simulink model "RLC_embedded_coder"  (R2022b)
settings: Solver=FixedStepDiscrete  StartTime=0.0  StopTime=Inf  RelTol=1e-3
InitFcn:
  | parametri_embedded
undefined symbols (not defined in the file): ADC_gain, current_gain, current_offset, data_size, DiscIntNeverNeededParam, Down, GPTRIP1SEL, GPTRIP2SEL, i_max, Kd_u, Ki_i, Ki_u, Kp_i, Kp_u, offset_filter, PWM_PERIOD, ref_counter_cmpr, ref_counter_prd, ref_value_high, ref_value_low, SAMPLE_FREQ, SAMPLE_TIME, tau, TZ1, TZ2, u_max, Up, voltage_gain, voltage_offset
libraries: simulink x9, c2802xlib x3, c280xlib x2, c2000lib x1, c2806xlib x1
settings Model: SimulationMode=external  ExtModeTrigDuration=8  Creator=Jan  LastModifiedBy=Jan
settings SolverCC: ZeroCrossAlgorithm=Adaptive  AutoInsertRateTranBlk=on
settings DataIOCC: ReturnWorkspaceOutputs=off
settings OptimizationCC: UseDivisionForNetSlopeComputation=on  GainParamInheritBuiltInType=on  UseFloatMulNetSlope=on  DefaultUnderspecifiedDataType=single  PassReuseOutputArgsAs=Individual arguments  NoFixptDivByZeroProtection=on  EfficientFloat2IntCast=on  LifeSpan=1  MaxStackSize=1024  OptimizeBlockOrder=speed  DifferentSizesBufferReuse=on  DenormalBehavior=FlushToZero  EfficientTunableParamExpr=on
settings DebuggingCC: IgnoredZcDiagnostic=none  ParameterTunabilityLossMsg=error
settings HardwareCC: ProdBitPerChar=16  ProdBitPerInt=16  ProdBitPerPointer=32  ProdBitPerSizeT=32  ProdBitPerPtrDiffT=32  ProdLargestAtomicInteger=Integer  ProdLargestAtomicFloat=None  ProdWordSize=16  ProdLongLongMode=on  ProdHWDeviceType=Texas Instruments->C2000
settings SFSimCC: MATLABDynamicMemAlloc=off
settings RTWCC: Description=Embedded Coder  SystemTargetFile=ert.tlc  HardwareBoard=TI Piccolo F28069M LaunchPad  TLCOptions=-aInlineSetEventsForThisBaseRateFcn=TLC_FALSE -aSuppressMultiTaskScheduler=TLC_FALSE -aRateBasedStepFcn=1  TemplateMakefile=ert_default_tmf  Toolchain=Texas Instruments Code Composer Studio (C2000)
settings CodeAppCC: ForceParamTrailComments=on  IgnoreCustomStorageClasses=off  OperatorAnnotations=on  SimulinkDataObjDesc=on  SFDataObjDesc=on  CustomSymbolStrGlobalVar=rt$N$M  CustomSymbolStrType=$N$M  CustomSymbolStrFcn=$N$M$F  CustomSymbolStrMacro=$N$M  InsertBlockDesc=on
settings ERTTargetCC: CodeReplacementLibrary=TI C28x  IncludeMdlTerminateFcn=off  CombineSignalStateStructs=on  SupportComplex=off  SupportNonInlinedSFcns=on  ExtModeTransport=4  ExtModeStaticAlloc=on  ExtModeAutomaticAllocSize=off  ExtModeMexFile=ext_xcp  ExtModeIntrfLevel=Level2 - Open  ERTFilePackagingFormat=CompactWithDataFile

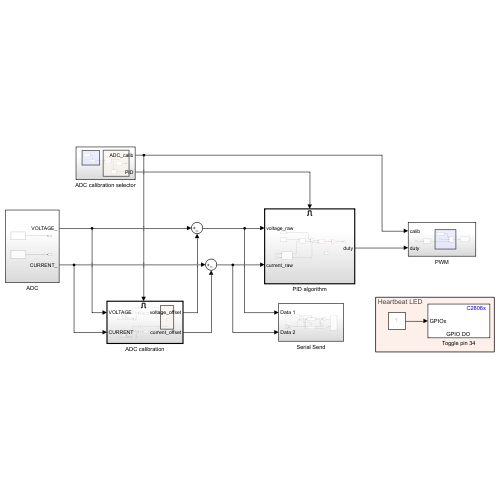
[thumbnail: Simulink's stored preview of the top-level diagram]
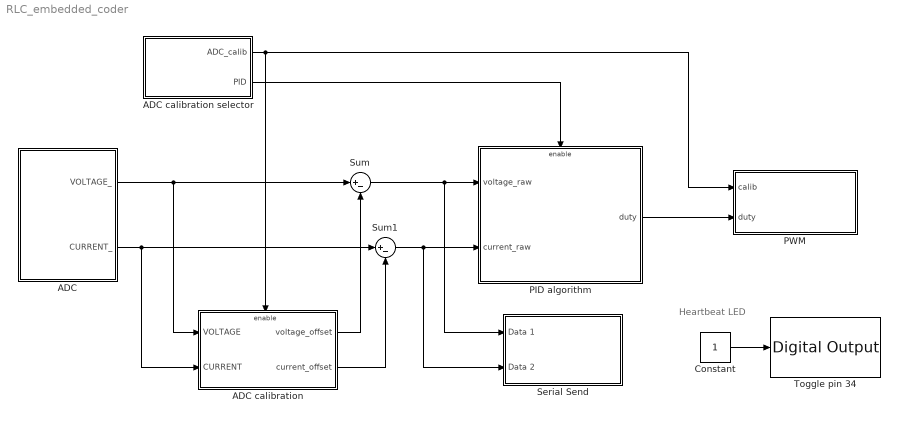
== system RLC_embedded_coder ==
  note: Heartbeat LED
  ADC : Subsystem
  ADC calibration : Subsystem
  ADC calibration selector : Subsystem
  Constant : Constant  SampleTime=0.7
  PID algorithm : Subsystem
  PWM : Subsystem
  Serial Send : Subsystem
  Sum : Sum  Inputs=|+-  OutDataTypeStr=Inherit: Same as first input
  Sum1 : Sum  Inputs=|+-  OutDataTypeStr=Inherit: Same as first input
  Toggle pin 34 : c2806xlib/Digital Output  GPIO_Number=GPIO32~GPIO39  GPIO_Bit0=off  GPIO_BIT0_Toggle=off  GPIO_Bit1=off  GPIO_BIT1_Toggle=off  GPIO_Bit2=on  GPIO_BIT2_Toggle=on  GPIO_Bit3=off  GPIO_BIT3_Toggle=off  GPIO_Bit4=off  GPIO_BIT4_Toggle=off  GPIO_Bit5=off  GPIO_BIT5_Toggle=off  GPIO_Bit6=off  GPIO_BIT6_Toggle=off  GPIO_Bit7=off  GPIO_BIT7_Toggle=off
  wires:
  Constant/1 -> Toggle pin 34/1
  ADC/2(CURRENT_) -> ADC calibration/2(CURRENT), Sum1/1
  ADC calibration selector/2(PID) -> PID algorithm/Enable
  Sum/1 -> Serial Send/1(Data 1), PID algorithm/1(voltage_raw)
  Sum1/1 -> PID algorithm/2(current_raw), Serial Send/2(Data 2)
  ADC/1(VOLTAGE_) -> ADC calibration/1(VOLTAGE), Sum/1
  PID algorithm/1(duty) -> PWM/2(duty)
  ADC calibration/1(voltage_offset) -> Sum/2
  ADC calibration/2(current_offset) -> Sum1/2
  ADC calibration selector/1(ADC_calib) -> PWM/1(calib), ADC calibration/Enable

== system RLC_embedded_coder/ADC ==
  note: ADC
  CURRENT : c2802xlib/ADC  blkParamProc=C2000  ADCModule=1  samplingMode=Single sample mode  ADCResolution=12-bit (Single-ended input)  useSOC1=SOC2  useSOC2=SOC0_SOC1  SOCAcquisitionWindow=7  SOCTriggerSource=ePWM1_ADCSOCA  SOCInterruptTrigger=No ADCINT  Ts=SAMPLE_TIME  dType=int16  postInterrupt=on  interruptSel=ADCINT1  ADCINTContinuous=off  endma=off  chdma=1  conv1=ADCINA0  conv2=ADCINA0 and ADCINB0  conv1_Type4=ADCIN0  conv2_Type4=ADCIN0 and ADCIN1
      settings: LibrarySourceBlock=c2806xlib/ADC
  VOLTAGE : c2802xlib/ADC  blkParamProc=C2000  ADCModule=1  samplingMode=Single sample mode  ADCResolution=12-bit (Single-ended input)  useSOC1=SOC1  useSOC2=SOC0_SOC1  SOCAcquisitionWindow=7  SOCTriggerSource=ePWM1_ADCSOCA  SOCInterruptTrigger=No ADCINT  Ts=SAMPLE_TIME  dType=int16  postInterrupt=off  interruptSel=ADCINT1  ADCINTContinuous=off  endma=off  chdma=1  conv1=ADCINA1  conv2=ADCINA0 and ADCINB0  conv1_Type4=ADCIN0  conv2_Type4=ADCIN0 and ADCIN1
      settings: LibrarySourceBlock=c2806xlib/ADC
  VOLTAGE_ : Outport
  CURRENT_ : Outport  Port=2
  wires:
  VOLTAGE/1 -> VOLTAGE_/1
  CURRENT/1 -> CURRENT_/1

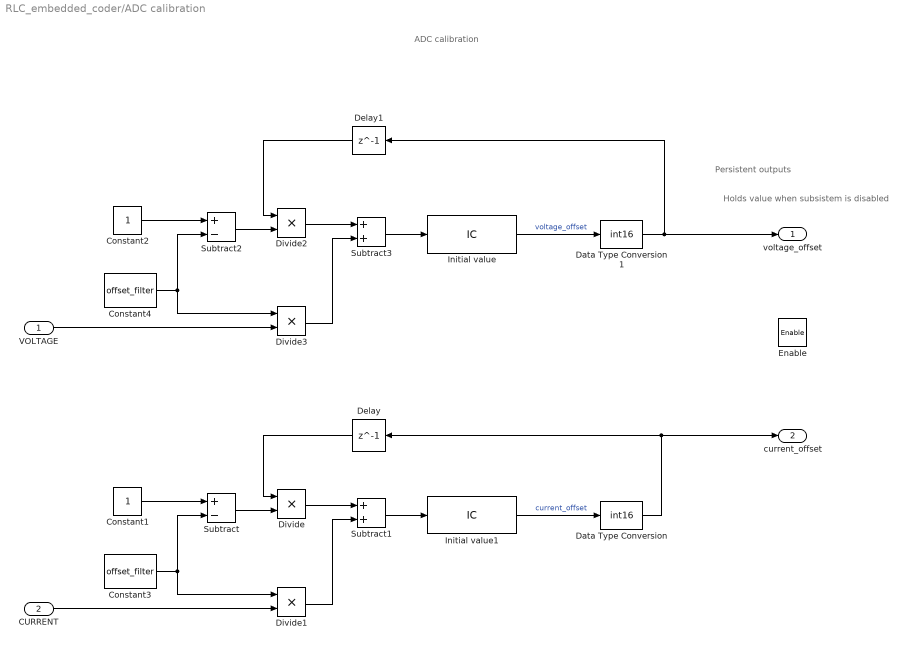
== system RLC_embedded_coder/ADC calibration ==
  note: Holds value when subsistem is disabled
  note: Persistent outputs
  note: ADC calibration
  VOLTAGE : Inport
  CURRENT : Inport  Port=2
  Enable : EnablePort
  Constant1 : Constant
  Constant2 : Constant
  Constant3 : Constant  Value=offset_filter
  Constant4 : Constant  Value=offset_filter
  Data Type Conversion : DataTypeConversion  OutDataTypeStr=int16  SaturateOnIntegerOverflow=off  RndMeth=Floor
  Data Type Conversion1 : DataTypeConversion  OutDataTypeStr=int16  SaturateOnIntegerOverflow=off  RndMeth=Floor
  Delay : Delay  DelayLength=1
  Delay1 : Delay  DelayLength=1
  Divide{,1..3} (4 alike) : Product  Inputs=**
  Initial value : InitialCondition  Value=voltage_offset
  Initial value1 : InitialCondition  Value=current_offset
  Subtract : Sum  Inputs=+-
  Subtract1 : Sum
  Subtract2 : Sum  Inputs=+-
  Subtract3 : Sum
  voltage_offset : Outport  OutDataTypeStr=int16
  current_offset : Outport  Port=2  OutDataTypeStr=int16
  wires:
  Subtract/1 -> Divide/2
  CURRENT/1 -> Divide1/2
  Constant3/1 -> Subtract/2, Divide1/1
  Constant1/1 -> Subtract/1
  Divide/1 -> Subtract1/1
  Divide1/1 -> Subtract1/2
  Delay/1 -> Divide/1
  Data Type Conversion/1 -> current_offset/1, Delay/1
  Delay1/1 -> Divide2/1
  Divide3/1 -> Subtract3/2
  Constant2/1 -> Subtract2/1
  VOLTAGE/1 -> Divide3/2
  Divide2/1 -> Subtract3/1
  Constant4/1 -> Subtract2/2, Divide3/1
  Subtract2/1 -> Divide2/2
  Initial value/1 -> Data Type Conversion1/1  "voltage_offset"
  Subtract3/1 -> Initial value/1
  Data Type Conversion1/1 -> voltage_offset/1, Delay1/1
  Subtract1/1 -> Initial value1/1
  Initial value1/1 -> Data Type Conversion/1  "current_offset"

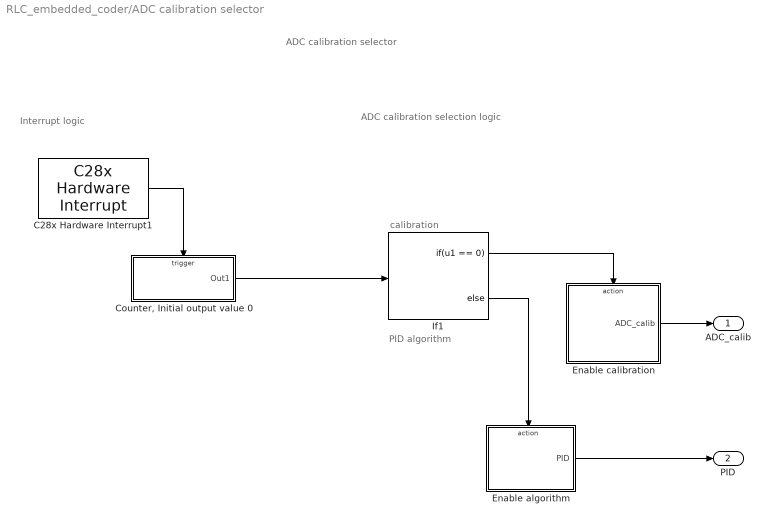
== system RLC_embedded_coder/ADC calibration selector ==
  note: calibration
  note: ADC calibration selection logic
  note: Interrupt logic
  note: PID algorithm
  note: ADC calibration selector
  C28x Hardware Interrupt1 : c2000lib/Scheduling/C28x Hardware Interrupt  irqnumbers=1  pienumbers=4  irqpriorities=30  irqpreempts=1  showinput=off  dspchiptype=C280X
  "Counter, Initial output value 0" : Subsystem  TreatAsAtomicUnit=on
  Enable algorithm : Subsystem  TreatAsAtomicUnit=on
  Enable calibration : Subsystem  TreatAsAtomicUnit=on
  If1 : If  IfExpression=u1 == 0
  ADC_calib : Outport
  PID : Outport  Port=2
  wires:
  If1/1 -> Enable calibration/Action
  If1/2 -> Enable algorithm/Action
  Enable algorithm/1(PID) -> PID/1
  Enable calibration/1(ADC_calib) -> ADC_calib/1
  C28x Hardware Interrupt1/1 -> "Counter, Initial output value 0"/Trigger
  "Counter, Initial output value 0"/1(Out1) -> If1/1

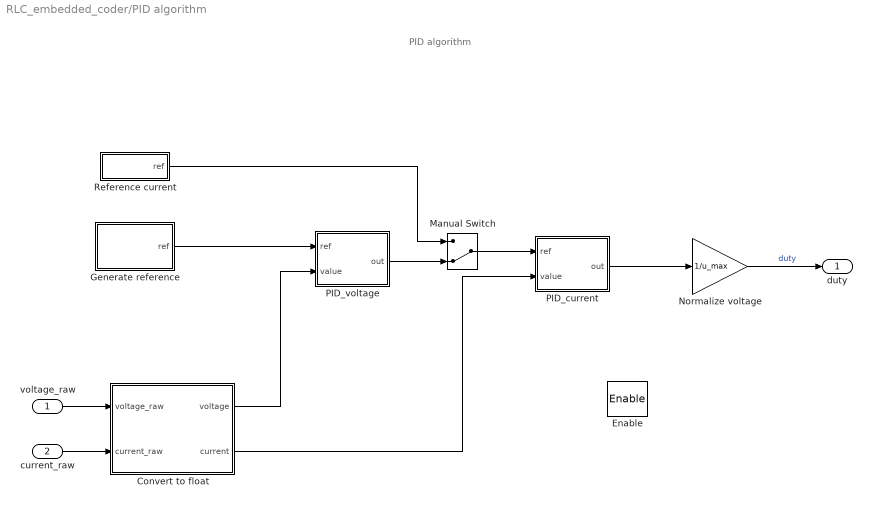
== system RLC_embedded_coder/PID algorithm ==
  note: PID algorithm
  voltage_raw : Inport
  current_raw : Inport  Port=2
  Enable : EnablePort
  Convert to float : Subsystem
  Generate reference : Subsystem
  Manual Switch : ManualSwitch  CurrentSetting=0
  Normalize voltage : Gain  Gain=1/u_max
  PID_current : Subsystem  mask{Kp=Kp_i, Ki=Ki_i, Kd=0, tau=0, lim=u_max, SAMPLE_TIME=SAMPLE_TIME}
      mask prompts: Kp "Proportional Gain"; Ki "Integral Gain"; Kd "Derivative Gain"; tau "Derivative filter"; lim "Output Limit"; SAMPLE_TIME "Sample Time"
      mask DialogControl DescTextVar Prompt: Discrete PID controller with D term filtering
  PID_voltage : Subsystem  mask{Kp=Kp_u, Ki=Ki_u, Kd=Kd_u, tau=tau, lim=i_max, SAMPLE_TIME=SAMPLE_TIME}
      mask prompts: Kp "Proportional Gain"; Ki "Integral Gain"; Kd "Derivative Gain"; tau "Derivative filter"; lim "Output Limit"; SAMPLE_TIME "Sample Time"
      mask DialogControl DescTextVar Prompt: Discrete PID controller with D term filtering
  Reference current : Subsystem
  duty : Outport
  wires:
  Generate reference/1(ref) -> PID_voltage/1(ref)
  Reference current/1(ref) -> Manual Switch/1
  Manual Switch/1 -> PID_current/1(ref)
  PID_voltage/1(out) -> Manual Switch/2
  PID_current/1(out) -> Normalize voltage/1
  Normalize voltage/1 -> duty/1  "duty"
  voltage_raw/1 -> Convert to float/1(voltage_raw)
  current_raw/1 -> Convert to float/2(current_raw)
  Convert to float/1(voltage) -> PID_voltage/2(value)
  Convert to float/2(current) -> PID_current/2(value)

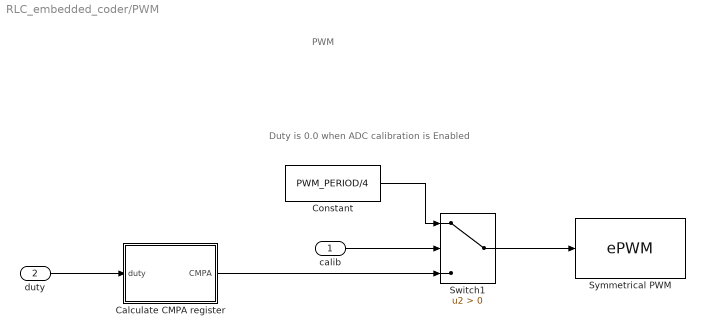
== system RLC_embedded_coder/PWM ==
  note: Duty is 0.0 when ADC calibration is Enabled
  note: PWM
  calib : Inport
  duty : Inport  Port=2
  Calculate CMPA register : Subsystem
  Constant : Constant  Value=PWM_PERIOD/4  SampleTime=-1
  Switch1 : Switch  Criteria=u2 > Threshold  SaturateOnIntegerOverflow=off  InputSameDT=off
  Symmetrical PWM : c2802xlib/ePWM  PwmType=C2000  useModule=ePWM1  ePWMxLINKTBPRD=Not Linked  periodUnits=Clock cycles  timerSource=Specify via dialog  timerPeriod_clk=int32(PWM_PERIOD/2)  timerPeriod_sec=0.0001  tbshadow=Counter equals to zero  countingMode=Up-Down  phaseActiveEnable=Disable  phaseDirection=Count down after sync  phaseActive=0  synchronizationEnable=off  dcaevt1Sync=off  dcbevt1Sync=off  synchronizationOption=Disable  dcbevt1SyncOut=off  dcaevt1SyncOut=off  cmpdSyncOut=off  cmpcSyncOut=off  cmpbSyncOut=off  zeroSyncOut=off  swfSyncOut=off  perSynchronizationOption=Counter equals to period (CTR=PRD)  clockPrescale=1  HSclockPrescale=1  enswap=off  ePWMxAStatus=on  ePWMxAactionLogic1=Do nothing  ePWMxAactionLogic2=Do nothing  ePWMxAactionLogic3=Set  ePWMxAactionLogic4=Clear  ePWMxAactionLogic5=Do nothing  ePWMxAactionLogic6=Do nothing  ePWMxACSFenable=off  ePWMxACSFvalue=Forcing disable  ePWMxASFreload=Zero  ePWMxBStatus=on  ePWMxBactionLogic1=Do nothing  ePWMxBactionLogic2=Do nothing  ePWMxBactionLogic3=Clear  ePWMxBactionLogic4=Set  ePWMxBactionLogic5=Do nothing  ePWMxBactionLogic6=Do nothing  ePWMxBCSFenable=off  ePWMxBCSFvalue=Forcing disable  ePWMxBSFreload=Zero  ePWNxBOutWay=on  ePWMxLINKCMPA=Not Linked  CMPAUnits=Clock cycles  CMPASource=Input port  CMPAValue_per=0  CMPAValue_clk=0  enCMPAshadow=Counter equals to zero (CTR=Zero)  ePWMxLINKCMPB=Not Linked  CMPBUnits=Clock cycles  CMPBSource=Specify via dialog  CMPBValue_per=0  CMPBValue_clk=0  enCMPBshadow=Counter equals to zero (CTR=Zero)  ePWMxLINKCMPC=Not Linked  CMPCUnits=Clock cycles  CMPCSource=Specify via dialog  CMPCValue_per=50  CMPCValue_clk=32000  enCMPCshadow=Counter equals to zero (CTR=Zero)  ePWMxLINKCMPD=Not Linked  CMPDUnits=Clock cycles  CMPDSource=Specify via dialog  CMPDValue_per=50  CMPDValue_clk=32000  enCMPDshadow=Counter equals to zero (CTR=Zero)  enableDBePWMxA=off  enableDBePWMxB=off  enhalfcycle=off  DBpolarity=Active high (AH)  DBedgeDelay=Positive  DBSource_ePWMxA=ePWMxA  DBSource_ePWMxB=ePWMxA  DBPeriodUnits=Clock cycles  DBperiodSource=Specify via dialog  REDperiod=0  FEDperiod=0  REDperiod_sec=0  FEDperiod_sec=0  LoadModeDBRED=Immediate without using shadow  LoadModeDBFED=Immediate without using shadow  adcstartModuleA=on  adcrequestEventA=First event  adcstartEventA=Counter equals to zero (CTR=Zero)  adcstartEventA_type2=Digital Compare Module A Event 1 start of conversion (DCAEVT1.soc)  adcstartModuleB=off  adcrequestEventB=First event  adcstartEventB=Counter equals to zero (CTR=Zero)  adcstartEventB_type2=Counter equals to zero (CTR=Zero)  intEn=off  intPrd=First event  intSel=Counter equals to zero (CTR=Zero)  intSel_type2=Counter equals to zero (CTR=Zero)  hrpe=off  enHRPWM=off  HRPWM_LoadMode=Counter equals to period (CTR=PRD)  HRPWM_CTLMode=Duty or Period control mode  HRPWM_EDGMode=Both edge  hrpeb=off  enHRPWMB=off  HRPWM_LoadModeB=Counter equals to zero (CTR=ZERO)  HRPWM_CTLModeB=Duty or Period control mode  HRPWM_EDGModeB=Both edge  enHRDBRED=off  enHRDBFED=off  enSFO=on  enautoconv=on  chopperEnable=off  chopperFrequency=1  chopperFirstwidth=1  chopperDuty=12.5%  tripZonesource=Specify via dialog  tzselOSHT1=off  tzselOSHT2=off  tzselOSHT3=off  tzselOSHDCAEV1=off  tzselOSHDCBEV1=off  tzselCBC1=off  tzselCBC2=off  tzselCBC3=off  tzselCBCDCAEV2=off  tzselCBCDCBEV2=off  tzselOSHT4=off  tzselOSHT5=off  tzselOSHT6=off  tzselCBC4=off  tzselCBC5=off  tzselCBC6=off  enTzOstIntr=off  enTzCbcIntr=off  enTzDCAEVT1Intr=off  enTzDCAEVT2Intr=off  enTzDCBEVT1Intr=off  enTzDCBEVT2Intr=off  ePWMxAforced=No action  ePWMxBforced=No action  DCAEVT1forced=No action  DCBEVT1forced=No action  DCAEVT2forced=No action  DCBEVT2forced=No action  dcah=Trip Zone 1 input (TZ1)  dcal=Trip Zone 2 input (TZ2)  dcbh=Trip Zone 1 input (TZ1)  dcbl=Trip Zone 2 input (TZ2)  dcah_type2=GPTRIP1SEL/(TZ1)  dcal_type2=GPTRIP2SEL/(TZ2)  dcbh_type2=GPTRIP1SEL/(TZ1)  dcbl_type2=GPTRIP2SEL/(TZ2)  gendcaevt1=Event disabled  gendcaevt2=Event disabled  gendcbevt1=Event disabled  gendcbevt2=Event disabled  dcaevt1src=DCAEVT1 with sync  dcaevt2src=DCAEVT2 with sync  dcbevt1src=DCBEVT1 with sync  dcbevt2src=DCBEVT2 with sync  pulsesel=Counter equals to zero (CTR=Zero)  blankinv=off  blankoffset=0  blankwidth=0  evsrcsel=Filtered version of DCAEVT1 (DCAEVT1FILT)  encape=off
      settings: LibrarySourceBlock=c2806xlib/ePWM
  wires:
  Switch1/1 -> Symmetrical PWM/1
  Calculate CMPA register/1(CMPA) -> Switch1/3
  calib/1 -> Switch1/2
  Constant/1 -> Switch1/1
  duty/1 -> Calculate CMPA register/1(duty)

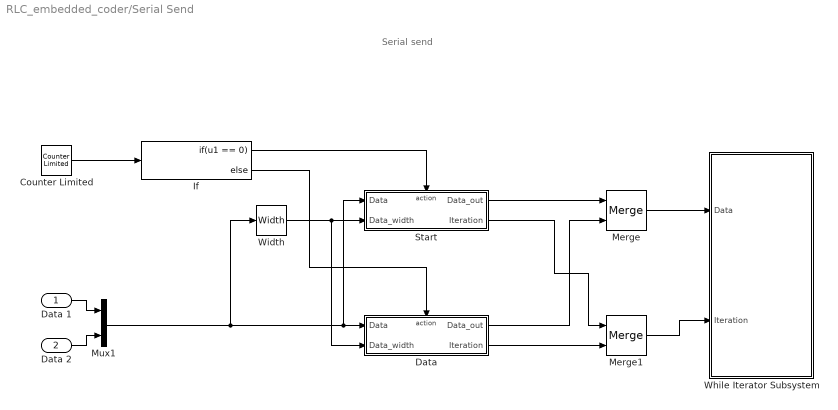
== system RLC_embedded_coder/Serial Send ==
  note: Serial send
  Data 1 : Inport
  Data 2 : Inport  Port=2
  Counter Limited : simulink/Sources/Counter Limited  uplimit=data_size-1  tsamp=-1
  Data : Subsystem  TreatAsAtomicUnit=on
  If : If  IfExpression=u1 == 0
  Merge : Merge
  Merge1 : Merge
  Mux1 : Mux  Inputs=2
  Start : Subsystem  TreatAsAtomicUnit=on
  While Iterator Subsystem : Subsystem  TreatAsAtomicUnit=on
  Width : Width  OutDataTypeMode=All ports same datatype  DataType=uint16
  wires:
  If/1 -> Start/Action
  If/2 -> Data/Action
  Counter Limited/1 -> If/1
  Start/1(Data_out) -> Merge/1
  Data/1(Data_out) -> Merge/2
  Merge/1 -> While Iterator Subsystem/1(Data)
  Merge1/1 -> While Iterator Subsystem/2(Iteration)
  Start/2(Iteration) -> Merge1/1
  Data/2(Iteration) -> Merge1/2
  Width/1 -> Data/2(Data_width), Start/2(Data_width)
  Mux1/1 -> Width/1, Start/1(Data), Data/1(Data)
  Data 1/1 -> Mux1/1
  Data 2/1 -> Mux1/2

== system RLC_embedded_coder/ADC calibration selector/Counter, Initial output value 0 ==
  note: ADC calibration counter
  function : TriggerPort  TriggerType=function-call  VariantControl=(inherit)
  Compare To Constant : simulink/Logic and Bit Operations/Compare To Constant  relop=>=  const=5*SAMPLE_FREQ  OutDataTypeStr=uint8
  Counter Free-Running : simulink/Sources/Counter Free-Running  NumBits=32  tsamp=-1
  Out1 : Outport  InitialOutput=[0]
  wires:
  Counter Free-Running/1 -> Compare To Constant/1
  Compare To Constant/1 -> Out1/1

== system RLC_embedded_coder/ADC calibration selector/Enable algorithm ==
  note: Enable algorithm
  Action Port : ActionPort  ActionPortLabel=else
  Constant : Constant
  PID : Outport  OutputWhenDisabled=reset  InitialOutput=[0]
  wires:
  Constant/1 -> PID/1

== system RLC_embedded_coder/ADC calibration selector/Enable calibration ==
  note: Enable calibration
  note: Trigger interrupt to disable ADC calibration
  Action Port : ActionPort  ActionPortLabel=if(u1 == 0)
  Constant : Constant
  Software Interrupt Trigger : c280xlib/Software Interrupt Trigger  irqnumbers=1  pienumbers=4  triggervalue=0  dspchiptype=C280X
      settings: LibrarySourceBlock=c2806xlib/Software Interrupt Trigger
  ADC_calib : Outport  OutputWhenDisabled=reset  InitialOutput=[0]
  wires:
  Constant/1 -> ADC_calib/1, Software Interrupt Trigger/1

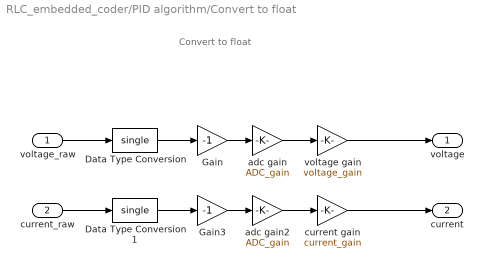
== system RLC_embedded_coder/PID algorithm/Convert to float ==
  note: Convert to float
  voltage_raw : Inport
  current_raw : Inport  Port=2
  Data Type Conversion : DataTypeConversion  OutDataTypeStr=single  SaturateOnIntegerOverflow=off  RndMeth=Floor
  Data Type Conversion1 : DataTypeConversion  OutDataTypeStr=single  SaturateOnIntegerOverflow=off  RndMeth=Floor
  Gain : Gain  Gain=-1
  Gain3 : Gain  Gain=-1
  adc gain : Gain  Gain=ADC_gain
  adc gain2 : Gain  Gain=ADC_gain
  current gain : Gain  Gain=current_gain
  voltage gain : Gain  Gain=voltage_gain
  voltage : Outport
  current : Outport  Port=2
  wires:
  Data Type Conversion/1 -> Gain/1
  adc gain/1 -> voltage gain/1
  Gain/1 -> adc gain/1
  voltage gain/1 -> voltage/1
  adc gain2/1 -> current gain/1
  Data Type Conversion1/1 -> Gain3/1
  Gain3/1 -> adc gain2/1
  current_raw/1 -> Data Type Conversion1/1
  voltage_raw/1 -> Data Type Conversion/1
  current gain/1 -> current/1

== system RLC_embedded_coder/PID algorithm/Generate reference ==
  note: Generate voltage reference
  Compare To Constant : simulink/Logic and Bit Operations/Compare To Constant  relop=>=  const=ref_counter_cmpr  OutDataTypeStr=boolean
  Constant : Constant  Value=ref_value_high  SampleTime=-1
  Constant1 : Constant  Value=ref_value_low  SampleTime=-1
  Switch : Switch  Criteria=u2 > Threshold  SaturateOnIntegerOverflow=off  InputSameDT=off
  ref_period : simulink/Sources/Counter Limited  uplimit=ref_counter_prd  tsamp=-1
  ref : Outport
  wires:
  ref_period/1 -> Compare To Constant/1
  Compare To Constant/1 -> Switch/2
  Switch/1 -> ref/1
  Constant1/1 -> Switch/1
  Constant/1 -> Switch/3

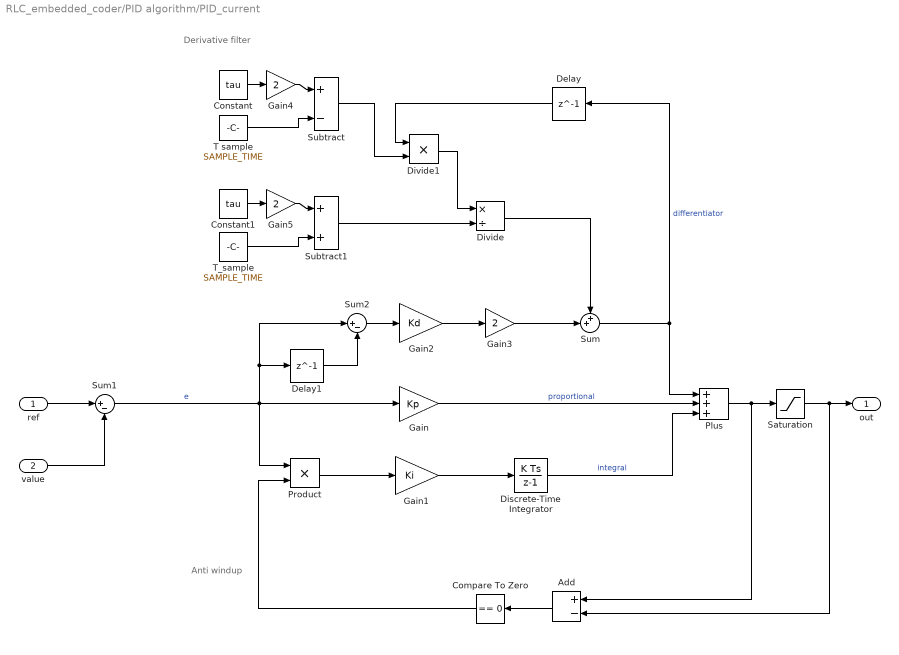
== system RLC_embedded_coder/PID algorithm/PID_current ==
  note: Derivative filter
  note: Anti windup
  ref : Inport
  value : Inport  Port=2
  Add : Sum  Inputs=+-
  Compare To Zero : simulink/Logic and Bit Operations/Compare To Zero  relop===  OutDataTypeStr=boolean
  Constant : Constant  Value=tau
  Constant1 : Constant  Value=tau
  Delay : Delay  DelayLength=1
  Delay1 : Delay  DelayLength=1
  Discrete-Time Integrator : DiscreteIntegrator  SampleTime=-1  ICPrevOutput=DiscIntNeverNeededParam  ICPrevScaledInput=DiscIntNeverNeededParam
  Divide : Product  Inputs=*/
  Divide1 : Product  Inputs=**
  Gain : Gain  Gain=Kp
  Gain1 : Gain  Gain=Ki
  Gain2 : Gain  Gain=Kd
  Gain3 : Gain  Gain=2
  Gain4 : Gain  Gain=2
  Gain5 : Gain  Gain=2
  Plus : Sum  Inputs=+++
  Product : Product
  Saturation : Saturate  UpperLimit=lim  LowerLimit=-lim
  Subtract : Sum  Inputs=+-
  Subtract1 : Sum
  Sum : Sum  Inputs=++|
  Sum1 : Sum  Inputs=|+-
  Sum2 : Sum  Inputs=|+-
  T sample : Constant  Value=SAMPLE_TIME
  T_sample : Constant  Value=SAMPLE_TIME
  out : Outport
  wires:
  Plus/1 -> Add/1, Saturation/1
  Saturation/1 -> out/1, Add/2
  Add/1 -> Compare To Zero/1
  Product/1 -> Gain1/1
  Compare To Zero/1 -> Product/2
  Discrete-Time Integrator/1 -> Plus/3  "integral"
  ref/1 -> Sum1/1
  value/1 -> Sum1/2
  Gain1/1 -> Discrete-Time Integrator/1
  Gain/1 -> Plus/2  "proportional"
  Gain2/1 -> Gain3/1
  Sum/1 -> Plus/1, Delay/1  "differentiator"
  Constant/1 -> Gain4/1
  Gain4/1 -> Subtract/1
  T sample/1 -> Subtract/2
  Gain5/1 -> Subtract1/1
  T_sample/1 -> Subtract1/2
  Constant1/1 -> Gain5/1
  Subtract/1 -> Divide1/2
  Delay/1 -> Divide1/1
  Divide1/1 -> Divide/1
  Subtract1/1 -> Divide/2
  Divide/1 -> Sum/1
  Gain3/1 -> Sum/2
  Delay1/1 -> Sum2/2
  Sum1/1 -> Sum2/1, Delay1/1, Product/1, Gain/1  "e"
  Sum2/1 -> Gain2/1

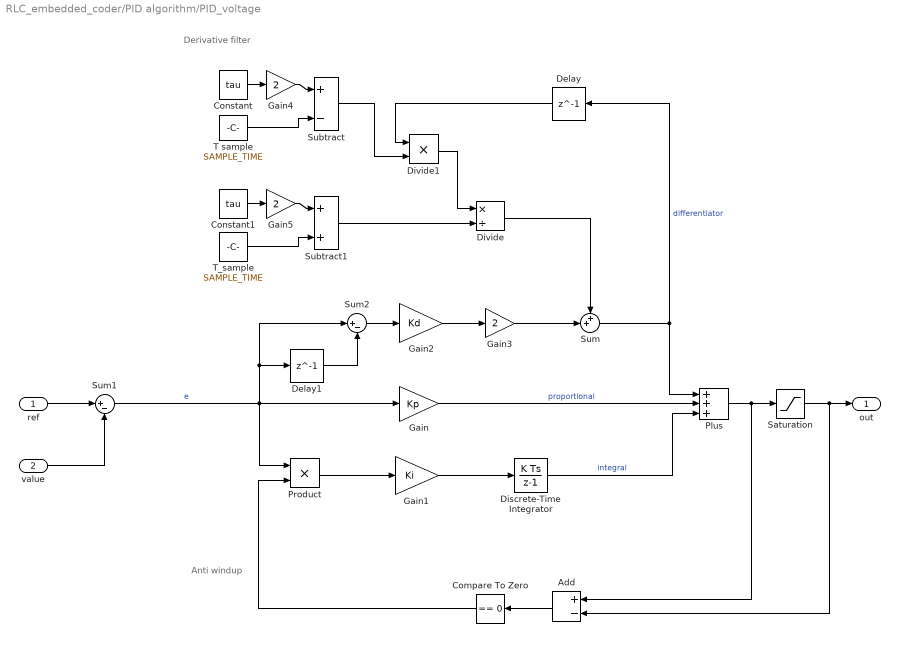
== system RLC_embedded_coder/PID algorithm/PID_voltage ==
  note: Derivative filter
  note: Anti windup
  ref : Inport
  value : Inport  Port=2
  Add : Sum  Inputs=+-
  Compare To Zero : simulink/Logic and Bit Operations/Compare To Zero  relop===  OutDataTypeStr=boolean
  Constant : Constant  Value=tau
  Constant1 : Constant  Value=tau
  Delay : Delay  DelayLength=1
  Delay1 : Delay  DelayLength=1
  Discrete-Time Integrator : DiscreteIntegrator  SampleTime=-1  ICPrevOutput=DiscIntNeverNeededParam  ICPrevScaledInput=DiscIntNeverNeededParam
  Divide : Product  Inputs=*/
  Divide1 : Product  Inputs=**
  Gain : Gain  Gain=Kp
  Gain1 : Gain  Gain=Ki
  Gain2 : Gain  Gain=Kd
  Gain3 : Gain  Gain=2
  Gain4 : Gain  Gain=2
  Gain5 : Gain  Gain=2
  Plus : Sum  Inputs=+++
  Product : Product
  Saturation : Saturate  UpperLimit=lim  LowerLimit=-lim
  Subtract : Sum  Inputs=+-
  Subtract1 : Sum
  Sum : Sum  Inputs=++|
  Sum1 : Sum  Inputs=|+-
  Sum2 : Sum  Inputs=|+-
  T sample : Constant  Value=SAMPLE_TIME
  T_sample : Constant  Value=SAMPLE_TIME
  out : Outport
  wires:
  Plus/1 -> Add/1, Saturation/1
  Saturation/1 -> out/1, Add/2
  Add/1 -> Compare To Zero/1
  Product/1 -> Gain1/1
  Compare To Zero/1 -> Product/2
  Discrete-Time Integrator/1 -> Plus/3  "integral"
  ref/1 -> Sum1/1
  value/1 -> Sum1/2
  Sum1/1 -> Sum2/1, Delay1/1, Product/1, Gain/1  "e"
  Gain1/1 -> Discrete-Time Integrator/1
  Gain/1 -> Plus/2  "proportional"
  Gain2/1 -> Gain3/1
  Sum/1 -> Plus/1, Delay/1  "differentiator"
  Constant/1 -> Gain4/1
  Gain4/1 -> Subtract/1
  T sample/1 -> Subtract/2
  Gain5/1 -> Subtract1/1
  T_sample/1 -> Subtract1/2
  Constant1/1 -> Gain5/1
  Subtract/1 -> Divide1/2
  Delay/1 -> Divide1/1
  Divide1/1 -> Divide/1
  Subtract1/1 -> Divide/2
  Divide/1 -> Sum/1
  Gain3/1 -> Sum/2
  Sum2/1 -> Gain2/1
  Delay1/1 -> Sum2/2

== system RLC_embedded_coder/PID algorithm/Reference current ==
  note: Generate current reference
  Compare To Constant : simulink/Logic and Bit Operations/Compare To Constant  relop=>=  const=20000  OutDataTypeStr=boolean
  Constant : Constant  Value=0  SampleTime=-1
  Constant1 : Constant  Value=4  SampleTime=-1
  Counter : simulink/Sources/Counter Limited  uplimit=ref_counter_prd  tsamp=-1
  Switch : Switch  Criteria=u2 > Threshold  SaturateOnIntegerOverflow=off  InputSameDT=off
  ref : Outport
  wires:
  Counter/1 -> Compare To Constant/1
  Compare To Constant/1 -> Switch/2
  Switch/1 -> ref/1
  Constant1/1 -> Switch/1
  Constant/1 -> Switch/3

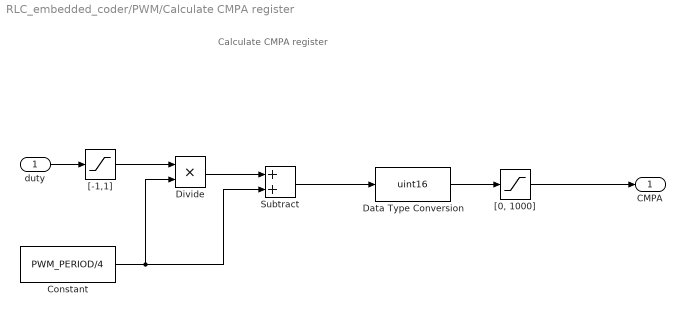
== system RLC_embedded_coder/PWM/Calculate CMPA register ==
  note: Calculate CMPA register
  duty : Inport
  Constant : Constant  Value=PWM_PERIOD/4  SampleTime=-1
  Data Type Conversion : DataTypeConversion  OutDataTypeStr=uint16  SaturateOnIntegerOverflow=off  RndMeth=Floor
  Divide : Product  Inputs=**
  Subtract : Sum
  "[-1,1]" : Saturate  UpperLimit=1  LowerLimit=-1
  "[0, 1000]" : Saturate  UpperLimit=PWM_PERIOD/2  LowerLimit=0
  CMPA : Outport
  wires:
  duty/1 -> "[-1,1]"/1
  Divide/1 -> Subtract/1
  Constant/1 -> Divide/2, Subtract/2
  "[-1,1]"/1 -> Divide/1
  Data Type Conversion/1 -> "[0, 1000]"/1
  Subtract/1 -> Data Type Conversion/1
  "[0, 1000]"/1 -> CMPA/1

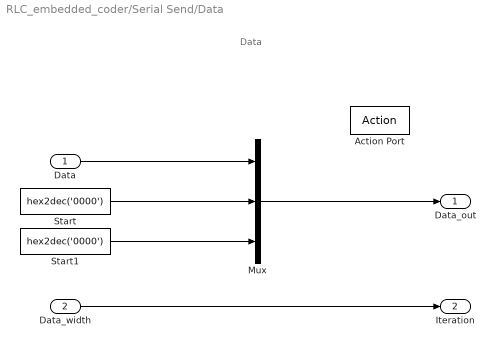
== system RLC_embedded_coder/Serial Send/Data ==
  note: Data
  Data : Inport
  Data_width : Inport  Port=2
  Action Port : ActionPort  ActionPortLabel=else
  Mux : Mux  Inputs=3
  Start : Constant  Value=hex2dec('0000')  OutDataTypeStr=int16
  Start1 : Constant  Value=hex2dec('0000')  OutDataTypeStr=int16
  Data_out : Outport
  Iteration : Outport  Port=2
  wires:
  Start/1 -> Mux/2
  Mux/1 -> Data_out/1
  Data/1 -> Mux/1
  Data_width/1 -> Iteration/1
  Start1/1 -> Mux/3

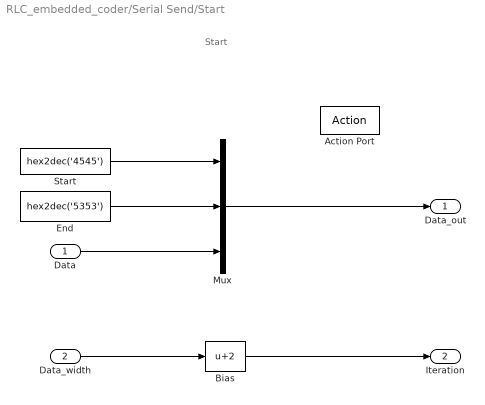
== system RLC_embedded_coder/Serial Send/Start ==
  note: Start
  Data : Inport
  Data_width : Inport  Port=2
  Action Port : ActionPort  ActionPortLabel=if(u1 == 0)
  Bias : Bias  Bias=2  SaturateOnIntegerOverflow=off
  End : Constant  Value=hex2dec('5353')  OutDataTypeStr=int16
  Mux : Mux  Inputs=3
  Start : Constant  Value=hex2dec('4545')  OutDataTypeStr=int16
  Data_out : Outport
  Iteration : Outport  Port=2
  wires:
  End/1 -> Mux/2
  Mux/1 -> Data_out/1
  Data_width/1 -> Bias/1
  Bias/1 -> Iteration/1
  Data/1 -> Mux/3
  Start/1 -> Mux/1

== system RLC_embedded_coder/Serial Send/While Iterator Subsystem ==
  note: Do-While
  Data : Inport
  Iteration : Inport  Port=2
  Add : Sum  Inputs=+-  OutDataTypeStr=Inherit: Same as first input
  Index Vector : MultiPortSwitch  Inputs=1  SaturateOnIntegerOverflow=off  InputSameDT=off
  SCI Transmit : c280xlib/SCI Transmit  sciModule=A  dataHead=''  dataTail=''  blockingMode=on  outputStatus=off
  While Iterator : WhileIterator  MaxIters=-1  WhileBlockType=do-while  ShowIterationPort=on  OutputDataType=int16
  wires:
  Iteration/1 -> Add/1
  Add/1 -> While Iterator/1
  Index Vector/1 -> SCI Transmit/1
  Data/1 -> Index Vector/2
  While Iterator/1 -> Index Vector/1, Add/2
